simulink model "GolfCartDCSeriesMotor"  (R2024b)
settings: Solver=VariableStepAuto  StartTime=0.0  StopTime=200  RelTol=1e-3
libraries: spsDCMachineLib x1, spsDCVoltageSourceLib x1, sps_lib x1
settings Model: Creator=brain  LastModifiedBy=brain

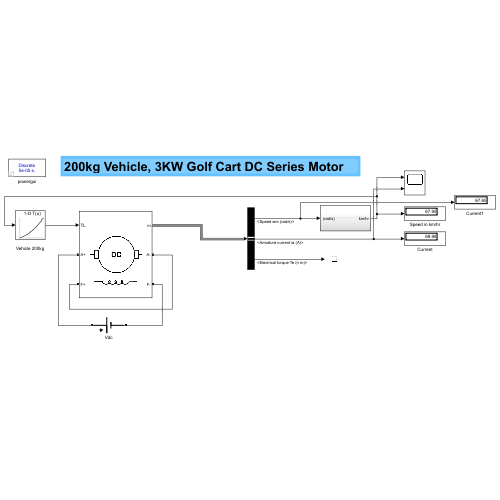
[thumbnail: Simulink's stored preview of the top-level diagram]
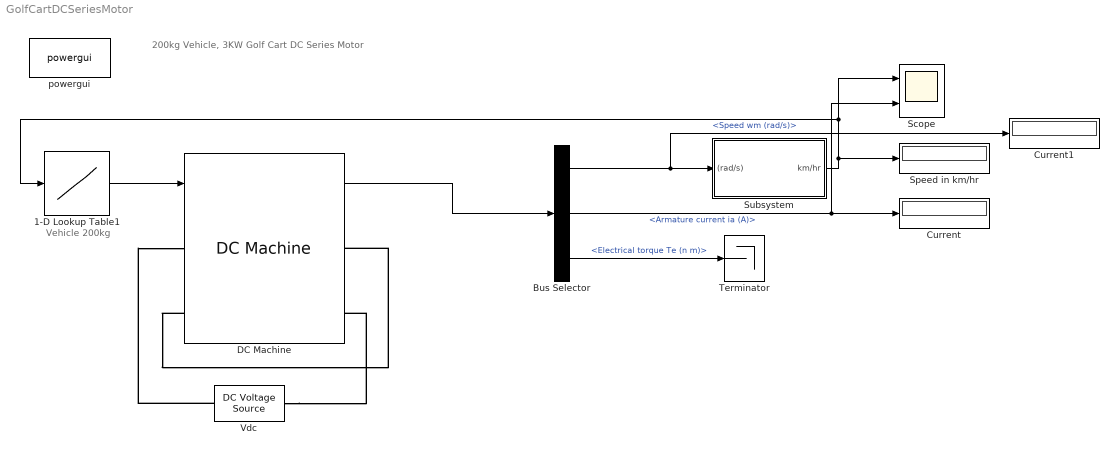
== system GolfCartDCSeriesMotor ==
  note: 200kg Vehicle, 3KW Golf Cart DC Series Motor
  note: Vehicle 200kg
  1-D Lookup Table1 : Lookup_n-D  NumberOfTableDimensions=1  BreakpointsForDimension1=[28.4 56.8 63.5 69.56 75.13 80.32 85.19 89.8 94.19 98.37 102.4 106.3 110 113.6 117.1 120.5 123.8 127]  Table=[5 20 25 30 35 40 45 50 55 60 65 70 75 80 85 90 95 100]  InternalRulePriority=Speed  RndMeth=Simplest
  Bus Selector : BusSelector  OutputSignals=Speed wm (rad/s),Armature current ia (A),Electrical torque Te (n m)
  Current : Display
  Current1 : Display
  DC Machine : spsDCMachineLib/DC Machine  PresetModel=No  MechanicalLoad=Torque TL  FieldType=Wound  ShowDetailedParameters=on  MeasurementBus=off  RLa="[ 0.18  0.00068]"  RLf="[ 0.1  0.0028]"  Laf=0.006  MachineConstant=Torque constant (N.m/A)  Ke=1.8  Kt=1.8  J=200*0.279*0.279  Bm=0.002953  Tf=0.5161  w0=1  Ifinit=171.428571428571  TsPowergui=0  TsBlock=-1
  Scope : Scope  NumInputPorts=2
  Speed in km/hr : Display
  Subsystem : Subsystem
  Terminator : Terminator
  Vdc : spsDCVoltageSourceLib/DC Voltage Source  Amplitude=48  Measurements=None
  powergui : sps_lib/powergui  Priority=1  SimulationMode=Discrete  SampleTime=50e-6  frequency=60  Iterations=50  frequencyindice=0  Pbase=100e6  ErrMax=1e-4  UnitsV=kV  UnitsW=MW  buscounter=0  FunctionMessages=off  echomessages=off  EnableUseOfTLC=off  CurrentSourceSwitches=off  DisableSnubberDevices=off  DisableRonSwitches=off  DisableVfSwitches=off  DisplayEquations=off  AutomaticDiscreteSolvers=off  SolverType=Tustin/Backward Euler (TBE)  Interpol=off  ExternalGateDelay=off  methode=off  Ts=100  x0status=blocks  SPID=on  SwTol=0  HookPort=off  NonlinearTolerance=1e-4  nMaxIteration=100  ContinueOnMaxIteration=off  RestoreLinks=warning  ResistiveCurrentMeasurement=off  Frange=[0:2:500]  Ylog=off  Xlog=on  ShowGrid=off  save=off  variable=ZData  structure=0  ZoomFFT=off  StartTime=0.0  cycles=1  DisplayStyle=1  fundamental=60  FreqAxis=off  MaxFrequency=1000  frequencyindicesteady=1  RmsSteady=1  display=off
  wires:
  Subsystem/1(km/hr) -> Scope/1, 1-D Lookup Table1/1, Speed in km/hr/1
  Bus Selector/1 -> Current1/1, Subsystem/1(" (rad/s)")  "<Speed wm (rad/s)>"
  Bus Selector/2 -> Scope/2, Current/1  "<Armature current ia (A)>"
  Bus Selector/3 -> Terminator/1  "<Electrical torque Te (n m)>"
  DC Machine/1 -> Bus Selector/1
  1-D Lookup Table1/1 -> DC Machine/1
  connections:
  Vdc/RConn1 -- DC Machine/LConn1
  Vdc/LConn1 -- DC Machine/RConn2
  DC Machine/LConn2 -- DC Machine/RConn1

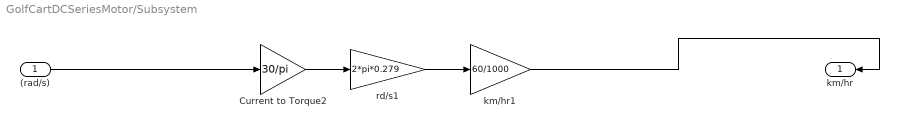
== system GolfCartDCSeriesMotor/Subsystem ==
  " (rad/s)" : Inport
  Current to Torque2 : Gain  Gain=30/pi
  km/hr1 : Gain  Gain=60/1000
  rd/s1 : Gain  Gain=2*pi*0.279
  km/hr : Outport
  wires:
  " (rad/s)"/1 -> Current to Torque2/1
  Current to Torque2/1 -> rd/s1/1
  rd/s1/1 -> km/hr1/1
  km/hr1/1 -> km/hr/1
